simulink model "InjCrv_PiIAddCor"  (R2016b)
settings: configuration reference "CodeGenConfigSet" (kept outside this file)
values from neighbouring files (symbols this model uses):
  InjCrv_phiPiI1StrtBase_MAP = Calibration.Parameter    [init_InjCrv_PiIAddCor.m]
  InjCrv_phiPiI1StrtBase_MAPX = Calibration.Parameter    [init_InjCrv_PiIAddCor.m]
  InjCrv_phiPiI1StrtBase_MAPY = Calibration.Parameter    [init_InjCrv_PiIAddCor.m]
  InjCrv_qPiI1StrtBase_MAP = Calibration.Parameter    [init_InjCrv_PiIAddCor.m]
  InjCrv_qPiI1StrtBase_MAPX = Calibration.Parameter    [init_InjCrv_PiIAddCor.m]
  InjCrv_qPiI1StrtBase_MAPY = Calibration.Parameter    [init_InjCrv_PiIAddCor.m]
  InjCrv_tiPiI1StrtBase_MAP = Calibration.Parameter    [init_InjCrv_PiIAddCor.m]
  InjCrv_tiPiI1StrtBase_MAPX = Calibration.Parameter    [init_InjCrv_PiIAddCor.m]
  InjCrv_tiPiI1StrtBase_MAPY = Calibration.Parameter    [init_InjCrv_PiIAddCor.m]
undefined symbols (not defined in the file or in its folder): EngState_conv
settings Model: Creator=Administrator  LastModifiedBy=wangrui
settings ConfigSetRef: SourceLocation=Base Workspace

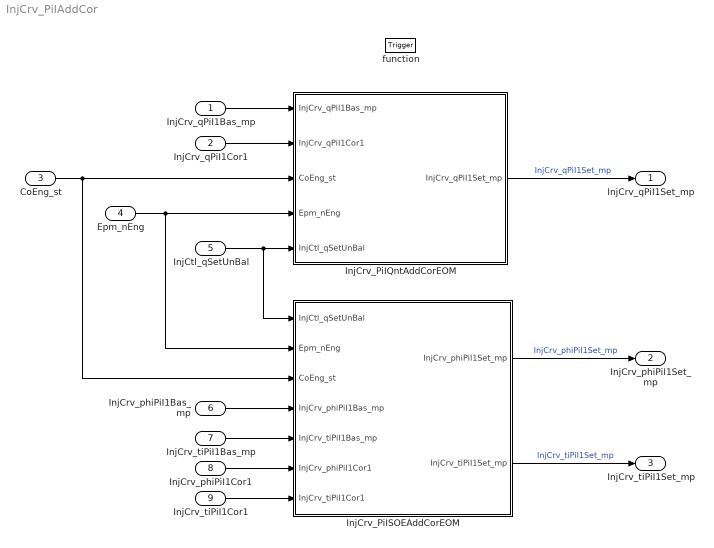
== system InjCrv_PiIAddCor ==
  InjCrv_qPiI1Bas_mp : Inport  Tag=mg/hub  Description=Basic injection quantity for PiI1  OutMin=-319  OutMax=319  OutDataTypeStr=FuelMass_mg_hub
  InjCrv_qPiI1Cor1 : Inport  Tag=mg/hub  Description=PiI quantity correction  Port=2  OutMin=-319  OutMax=319  OutDataTypeStr=FuelMass_mg_hub
  CoEng_st : Inport  Description=Engine coordinator state  Port=3  OutDataTypeStr=Enum: EngState_conv
  Epm_nEng : Inport  Tag=rpm  Description=Engine speed  Port=4  OutMin=0  OutMax=6000  OutDataTypeStr=EngSpeed_rpm
  InjCtl_qSetUnBal : Inport  Tag=mg/hub  Description=Current injection quantity  Port=5  OutMin=-319  OutMax=319  OutDataTypeStr=FuelMass_mg_hub
  InjCrv_phiPiI1Bas_mp : Inport  Tag=CA  Description=Basic PiI1 start of energizing(phi)  Port=6  OutMin=-719  OutMax=719  OutDataTypeStr=Angle_CA
  InjCrv_tiPiI1Bas_mp : Inport  Tag=us  Description=Basic PiI1 start of energizing(ti)  Port=7  OutMin=-13107  OutMax=13106  OutDataTypeStr=InjTime_us
  InjCrv_phiPiI1Cor1 : Inport  Tag=CA  Description=PiI1 start of energizing correction(phi)  Port=8  OutMin=-719  OutMax=719  OutDataTypeStr=Angle_CA
  InjCrv_tiPiI1Cor1 : Inport  Tag=us  Description=PiI1 start of energizing correction(ti)  Port=9  OutMin=-13107  OutMax=13106  OutDataTypeStr=InjTime_us
  function : TriggerPort  TriggerType=function-call  VariantControl=Variant
  InjCrv_PiIQntAddCorEOM : Subsystem  RTWFcnName=InjCrv_PiIQntAddCorEOM_Co  RTWFileName=InjCrv_PiIQntAddCorEOM
      settings: RTWSystemCode=Nonreusable function  RTWFcnNameOpts=User specified  RTWFileNameOpts=User specified
  InjCrv_PiISOEAddCorEOM : Subsystem  RTWFcnName=InjCrv_PiISOEAddCorEOM_Co  RTWFileName=InjCrv_PiISOEAddCorEOM
      settings: RTWSystemCode=Nonreusable function  RTWFcnNameOpts=User specified  RTWFileNameOpts=User specified
  InjCrv_qPiI1Set_mp : Outport  Tag=mg/hub  Description=Set PiI1 quantity  OutMin=-319  OutMax=319  OutDataTypeStr=FuelMass_mg_hub
  InjCrv_phiPiI1Set_mp : Outport  Tag=CA  Description=Set PiI1 start of energizing during starting time(phi)  Port=2  OutMin=-719  OutMax=719  OutDataTypeStr=Angle_CA
  InjCrv_tiPiI1Set_mp : Outport  Tag=us  Description=Set PiI1 start of energizing during starting time(ti)  Port=3  OutMin=-13107  OutMax=13106  OutDataTypeStr=InjTime_us
  wires:
  InjCrv_PiIQntAddCorEOM/1(InjCrv_qPiI1Set_mp) -> InjCrv_qPiI1Set_mp/1  "InjCrv_qPiI1Set_mp"
  InjCrv_PiISOEAddCorEOM/1(InjCrv_phiPiI1Set_mp) -> InjCrv_phiPiI1Set_mp/1  "InjCrv_phiPiI1Set_mp"
  InjCrv_PiISOEAddCorEOM/2(InjCrv_tiPiI1Set_mp) -> InjCrv_tiPiI1Set_mp/1  "InjCrv_tiPiI1Set_mp"
  InjCrv_qPiI1Bas_mp/1 -> InjCrv_PiIQntAddCorEOM/1(InjCrv_qPiI1Bas_mp)
  InjCrv_qPiI1Cor1/1 -> InjCrv_PiIQntAddCorEOM/2(InjCrv_qPiI1Cor1)
  Epm_nEng/1 -> InjCrv_PiIQntAddCorEOM/4(Epm_nEng), InjCrv_PiISOEAddCorEOM/2(Epm_nEng)
  InjCtl_qSetUnBal/1 -> InjCrv_PiIQntAddCorEOM/5(InjCtl_qSetUnBal), InjCrv_PiISOEAddCorEOM/1(InjCtl_qSetUnBal)
  InjCrv_phiPiI1Bas_mp/1 -> InjCrv_PiISOEAddCorEOM/4(InjCrv_phiPiI1Bas_mp)
  InjCrv_tiPiI1Bas_mp/1 -> InjCrv_PiISOEAddCorEOM/5(InjCrv_tiPiI1Bas_mp)
  InjCrv_phiPiI1Cor1/1 -> InjCrv_PiISOEAddCorEOM/6(InjCrv_phiPiI1Cor1)
  InjCrv_tiPiI1Cor1/1 -> InjCrv_PiISOEAddCorEOM/7(InjCrv_tiPiI1Cor1)
  CoEng_st/1 -> InjCrv_PiIQntAddCorEOM/3(CoEng_st), InjCrv_PiISOEAddCorEOM/3(CoEng_st)

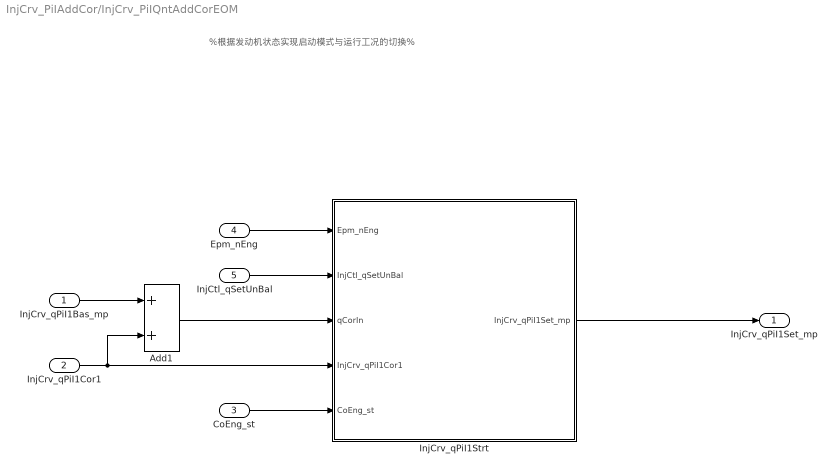
== system InjCrv_PiIAddCor/InjCrv_PiIQntAddCorEOM ==
  note: %根据发动机状态实现启动模式与运行工况的切换%
  InjCrv_qPiI1Bas_mp : Inport
  InjCrv_qPiI1Cor1 : Inport  Port=2
  CoEng_st : Inport  Port=3
  Epm_nEng : Inport  Port=4
  InjCtl_qSetUnBal : Inport  Port=5
  Add1 : Sum  InputSameDT=on
  InjCrv_qPiI1Strt : Subsystem
  InjCrv_qPiI1Set_mp : Outport
  wires:
  InjCrv_qPiI1Strt/1(InjCrv_qPiI1Set_mp) -> InjCrv_qPiI1Set_mp/1
  Add1/1 -> InjCrv_qPiI1Strt/3(qCorIn)
  InjCtl_qSetUnBal/1 -> InjCrv_qPiI1Strt/2(InjCtl_qSetUnBal)
  Epm_nEng/1 -> InjCrv_qPiI1Strt/1(Epm_nEng)
  CoEng_st/1 -> InjCrv_qPiI1Strt/5(CoEng_st)
  InjCrv_qPiI1Cor1/1 -> Add1/2, InjCrv_qPiI1Strt/4(InjCrv_qPiI1Cor1)
  InjCrv_qPiI1Bas_mp/1 -> Add1/1

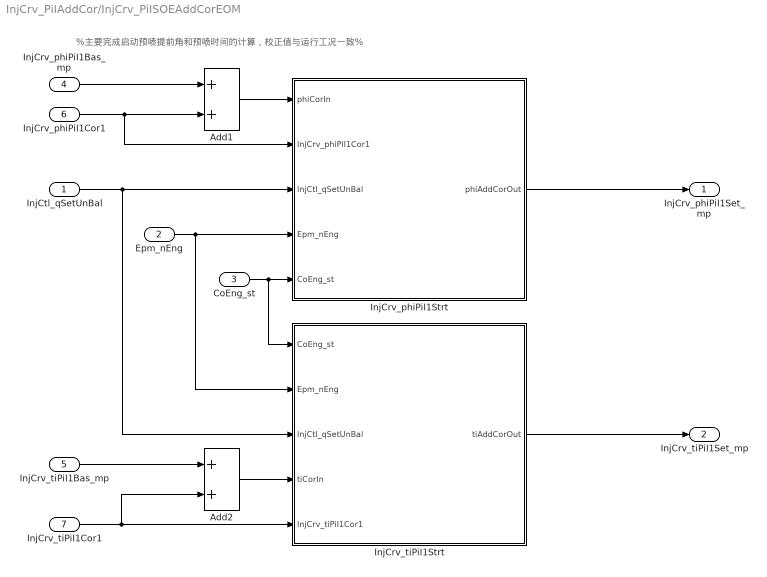
== system InjCrv_PiIAddCor/InjCrv_PiISOEAddCorEOM ==
  note: %主要完成启动预喷提前角和预喷时间的计算，校正值与运行工况一致%
  InjCtl_qSetUnBal : Inport
  Epm_nEng : Inport  Port=2
  CoEng_st : Inport  Port=3
  InjCrv_phiPiI1Bas_mp : Inport  Port=4
  InjCrv_tiPiI1Bas_mp : Inport  Port=5
  InjCrv_phiPiI1Cor1 : Inport  Port=6
  InjCrv_tiPiI1Cor1 : Inport  Port=7
  Add1 : Sum  InputSameDT=on
  Add2 : Sum  InputSameDT=on
  InjCrv_phiPiI1Strt : Subsystem
  InjCrv_tiPiI1Strt : Subsystem
  InjCrv_phiPiI1Set_mp : Outport
  InjCrv_tiPiI1Set_mp : Outport  Port=2
  wires:
  InjCrv_tiPiI1Strt/1(tiAddCorOut) -> InjCrv_tiPiI1Set_mp/1
  Add2/1 -> InjCrv_tiPiI1Strt/4(tiCorIn)
  InjCtl_qSetUnBal/1 -> InjCrv_phiPiI1Strt/3(InjCtl_qSetUnBal), InjCrv_tiPiI1Strt/3(InjCtl_qSetUnBal)
  Epm_nEng/1 -> InjCrv_phiPiI1Strt/4(Epm_nEng), InjCrv_tiPiI1Strt/2(Epm_nEng)
  CoEng_st/1 -> InjCrv_tiPiI1Strt/1(CoEng_st), InjCrv_phiPiI1Strt/5(CoEng_st)
  Add1/1 -> InjCrv_phiPiI1Strt/1(phiCorIn)
  InjCrv_phiPiI1Strt/1(phiAddCorOut) -> InjCrv_phiPiI1Set_mp/1
  InjCrv_tiPiI1Cor1/1 -> Add2/2, InjCrv_tiPiI1Strt/5(InjCrv_tiPiI1Cor1)
  InjCrv_tiPiI1Bas_mp/1 -> Add2/1
  InjCrv_phiPiI1Cor1/1 -> InjCrv_phiPiI1Strt/2(InjCrv_phiPiI1Cor1), Add1/2
  InjCrv_phiPiI1Bas_mp/1 -> Add1/1

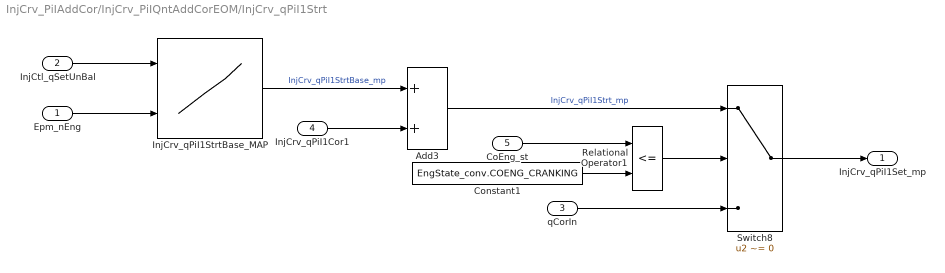
== system InjCrv_PiIAddCor/InjCrv_PiIQntAddCorEOM/InjCrv_qPiI1Strt ==
  Epm_nEng : Inport
  InjCtl_qSetUnBal : Inport  Port=2
  qCorIn : Inport  Port=3
  InjCrv_qPiI1Cor1 : Inport  Port=4
  CoEng_st : Inport  Port=5
  Add3 : Sum  InputSameDT=on
  Constant1 : Constant  Value=EngState_conv.COENG_CRANKING  OutDataTypeStr=Inherit: Inherit via back propagation
  InjCrv_qPiI1StrtBase_MAP : Lookup_n-D  BreakpointsForDimension1=InjCrv_qPiI1StrtBase_MAPY  BreakpointsForDimension2=InjCrv_qPiI1StrtBase_MAPX  IndexSearchMethod=Linear search  BeginIndexSearchUsingPreviousIndexResult=on  Table=InjCrv_qPiI1StrtBase_MAP  ExtrapMethod=Clip  UseLastTableValue=on  InternalRulePriority=Speed  OutDataTypeStr=Inherit: Inherit via back propagation  SaturateOnIntegerOverflow=on
  Relational Operator1 : RelationalOperator  Operator=<=  OutDataTypeStr=boolean  RndMeth=Nearest  InputSameDT=on
  Switch8 : Switch  Criteria=u2 ~= 0  InputSameDT=on
  InjCrv_qPiI1Set_mp : Outport
  wires:
  qCorIn/1 -> Switch8/3
  Switch8/1 -> InjCrv_qPiI1Set_mp/1
  CoEng_st/1 -> Relational Operator1/1
  Constant1/1 -> Relational Operator1/2
  Relational Operator1/1 -> Switch8/2
  Add3/1 -> Switch8/1  "InjCrv_qPiI1Strt_mp"
  InjCrv_qPiI1Cor1/1 -> Add3/2
  InjCrv_qPiI1StrtBase_MAP/1 -> Add3/1  "InjCrv_qPiI1StrtBase_mp"
  InjCtl_qSetUnBal/1 -> InjCrv_qPiI1StrtBase_MAP/1
  Epm_nEng/1 -> InjCrv_qPiI1StrtBase_MAP/2

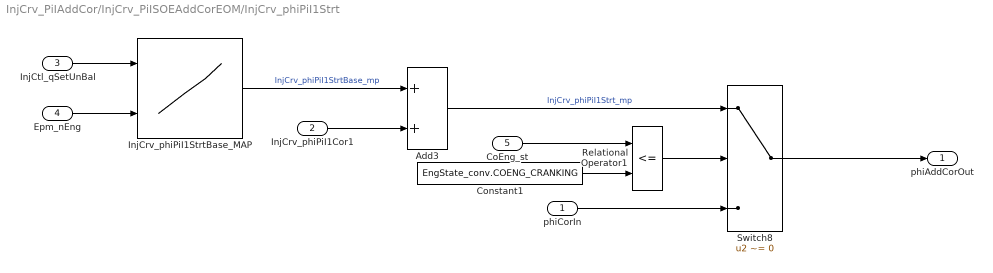
== system InjCrv_PiIAddCor/InjCrv_PiISOEAddCorEOM/InjCrv_phiPiI1Strt ==
  phiCorIn : Inport
  InjCrv_phiPiI1Cor1 : Inport  Port=2
  InjCtl_qSetUnBal : Inport  Port=3
  Epm_nEng : Inport  Port=4
  CoEng_st : Inport  Port=5
  Add3 : Sum  InputSameDT=on
  Constant1 : Constant  Value=EngState_conv.COENG_CRANKING  OutDataTypeStr=Inherit: Inherit via back propagation
  InjCrv_phiPiI1StrtBase_MAP : Lookup_n-D  BreakpointsForDimension1=InjCrv_phiPiI1StrtBase_MAPY  BreakpointsForDimension2=InjCrv_phiPiI1StrtBase_MAPX  IndexSearchMethod=Linear search  BeginIndexSearchUsingPreviousIndexResult=on  Table=InjCrv_phiPiI1StrtBase_MAP  ExtrapMethod=Clip  UseLastTableValue=on  InternalRulePriority=Speed  OutDataTypeStr=Inherit: Inherit via back propagation  SaturateOnIntegerOverflow=on
  Relational Operator1 : RelationalOperator  Operator=<=  OutDataTypeStr=boolean  RndMeth=Nearest  InputSameDT=on
  Switch8 : Switch  Criteria=u2 ~= 0  InputSameDT=on
  phiAddCorOut : Outport
  wires:
  phiCorIn/1 -> Switch8/3
  Switch8/1 -> phiAddCorOut/1
  CoEng_st/1 -> Relational Operator1/1
  Constant1/1 -> Relational Operator1/2
  Relational Operator1/1 -> Switch8/2
  Add3/1 -> Switch8/1  "InjCrv_phiPiI1Strt_mp"
  InjCrv_phiPiI1Cor1/1 -> Add3/2
  InjCrv_phiPiI1StrtBase_MAP/1 -> Add3/1  "InjCrv_phiPiI1StrtBase_mp"
  InjCtl_qSetUnBal/1 -> InjCrv_phiPiI1StrtBase_MAP/1
  Epm_nEng/1 -> InjCrv_phiPiI1StrtBase_MAP/2

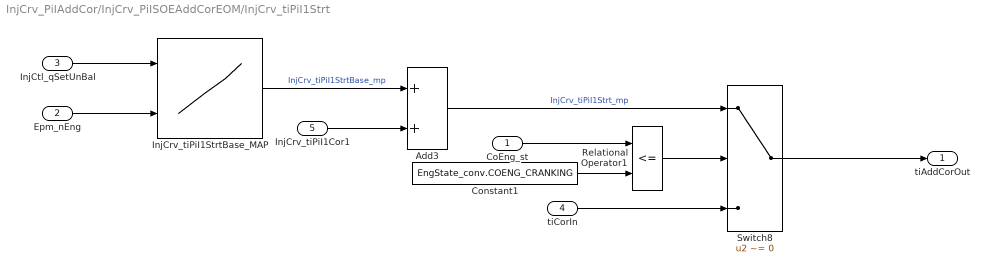
== system InjCrv_PiIAddCor/InjCrv_PiISOEAddCorEOM/InjCrv_tiPiI1Strt ==
  CoEng_st : Inport
  Epm_nEng : Inport  Port=2
  InjCtl_qSetUnBal : Inport  Port=3
  tiCorIn : Inport  Port=4
  InjCrv_tiPiI1Cor1 : Inport  Port=5
  Add3 : Sum  InputSameDT=on
  Constant1 : Constant  Value=EngState_conv.COENG_CRANKING  OutDataTypeStr=Inherit: Inherit via back propagation
  InjCrv_tiPiI1StrtBase_MAP : Lookup_n-D  BreakpointsForDimension1=InjCrv_tiPiI1StrtBase_MAPY  BreakpointsForDimension2=InjCrv_tiPiI1StrtBase_MAPX  IndexSearchMethod=Linear search  BeginIndexSearchUsingPreviousIndexResult=on  Table=InjCrv_tiPiI1StrtBase_MAP  ExtrapMethod=Clip  UseLastTableValue=on  InternalRulePriority=Speed  OutDataTypeStr=Inherit: Inherit via back propagation  SaturateOnIntegerOverflow=on
  Relational Operator1 : RelationalOperator  Operator=<=  OutDataTypeStr=boolean  RndMeth=Nearest  InputSameDT=on
  Switch8 : Switch  Criteria=u2 ~= 0  InputSameDT=on
  tiAddCorOut : Outport
  wires:
  Epm_nEng/1 -> InjCrv_tiPiI1StrtBase_MAP/2
  InjCtl_qSetUnBal/1 -> InjCrv_tiPiI1StrtBase_MAP/1
  InjCrv_tiPiI1StrtBase_MAP/1 -> Add3/1  "InjCrv_tiPiI1StrtBase_mp"
  InjCrv_tiPiI1Cor1/1 -> Add3/2
  Add3/1 -> Switch8/1  "InjCrv_tiPiI1Strt_mp"
  Relational Operator1/1 -> Switch8/2
  Constant1/1 -> Relational Operator1/2
  CoEng_st/1 -> Relational Operator1/1
  Switch8/1 -> tiAddCorOut/1
  tiCorIn/1 -> Switch8/3
